simulink model "Project1_1"  (R2015b)
settings: Solver=ode5  StartTime=0.0  StopTime=100  FixedStep=0.001  RelTol=1e-3
values from neighbouring files (symbols this model uses):
  x0 = 1    [Project1.m]
  x_dot0 = -2    [Project1.m]
settings Model: Creator=Dell  LastModifiedBy=Dell
settings DataIOCC: LimitDataPoints=off

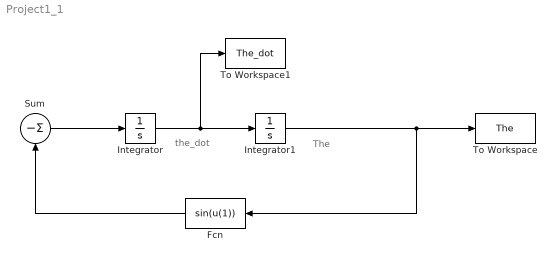
== system Project1_1 ==
  note: The
  note: the_dot
  Fcn : Fcn  Expr=sin(u(1))
  Integrator : Integrator  InitialCondition=x_dot0
  Integrator1 : Integrator  InitialCondition=x0
  Sum : Sum  Inputs=|-
  To Workspace : ToWorkspace  VariableName=The  SampleTime=-1
  To Workspace1 : ToWorkspace  VariableName=The_dot  SampleTime=-1
  wires:
  Sum/1 -> Integrator/1
  Integrator/1 -> To Workspace1/1, Integrator1/1
  Integrator1/1 -> Fcn/1, To Workspace/1
  Fcn/1 -> Sum/1
